simulink model "Problem_No4"  (R2020a)
settings: Solver=VariableStepAuto  StartTime=0.0  StopTime=10.0  RelTol=1e-3
settings Model: Creator='Z'ome  LastModifiedBy='Z'ome

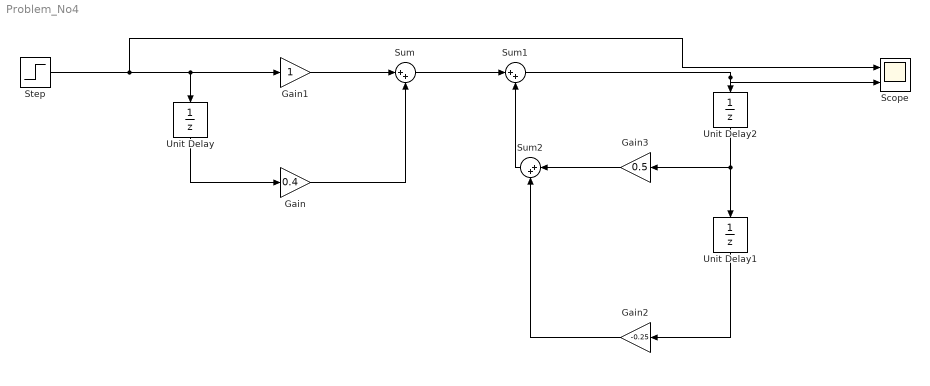
== system Problem_No4 ==
  Gain : Gain  Gain=0.4
  Gain1 : Gain
  Gain2 : Gain  Gain=-0.25
  Gain3 : Gain  Gain=0.5
  Scope : Scope  NumInputPorts=2
  Step : Step  SampleTime=0
  Sum : Sum  Inputs=|++
  Sum1 : Sum  Inputs=|++
  Sum2 : Sum  Inputs=|++
  Unit Delay : UnitDelay  SampleTime=-1  HasFrameUpgradeWarning=on
  Unit Delay1 : UnitDelay  SampleTime=-1  HasFrameUpgradeWarning=on
  Unit Delay2 : UnitDelay  SampleTime=-1  HasFrameUpgradeWarning=on
  wires:
  Unit Delay2/1 -> Gain3/1, Unit Delay1/1
  Unit Delay/1 -> Gain/1
  Step/1 -> Scope/1, Unit Delay/1, Gain1/1
  Gain/1 -> Sum/2
  Sum1/1 -> Unit Delay2/1, Scope/2
  Gain3/1 -> Sum2/1
  Gain1/1 -> Sum/1
  Sum/1 -> Sum1/1
  Gain2/1 -> Sum2/2
  Sum2/1 -> Sum1/2
  Unit Delay1/1 -> Gain2/1
